simulink model "msgOutPack"  (R2023b)
settings: Solver=FixedStepDiscrete  StartTime=0.0  StopTime=10.0  FixedStep=Ts_10ms  RelTol=1e-3  EnableMultiTasking=on
values from neighbouring files (symbols this model uses):
  Ts_10ms = 0.01    [msgOutPack.sldd]
libraries: canmsglib x1
settings Model: DataDictionary=msgOutPack.sldd  Creator=62555  LastModifiedBy=62555
settings DataIOCC: SaveOutput=off  SignalLogging=off  ReturnWorkspaceOutputs=off
settings OptimizationCC: DefaultParameterBehavior=Inlined  DefaultUnderspecifiedDataType=single  EnhancedBackFolding=on  PassReuseOutputArgsAs=Individual arguments  ZeroExternalMemoryAtStartup=off  ZeroInternalMemoryAtStartup=off  OptimizeBlockOrder=speed  DifferentSizesBufferReuse=on  OptimizationCustomize=off  EfficientTunableParamExpr=on
settings DebuggingCC: ParameterTunabilityLossMsg=error
settings HardwareCC: ProdBitPerPointer=32  ProdBitPerSizeT=32  ProdBitPerPtrDiffT=32  ProdLargestAtomicInteger=Long  ProdLargestAtomicFloat=Double  ProdWordSize=32  ProdHWDeviceType=ARM Compatible->ARM Cortex-M
settings SFSimCC: MATLABDynamicMemAlloc=off
settings RTWCC: Description=Embedded Coder  SystemTargetFile=ert.tlc  GenCodeOnly=on  TemplateMakefile=ert_default_tmf  GenerateReport=on  Toolchain=MinGW64 | gmake (64-bit Windows)
settings CodeAppCC: ForceParamTrailComments=on  IgnoreCustomStorageClasses=off  OperatorAnnotations=on  SimulinkDataObjDesc=on  SFDataObjDesc=on  InsertBlockDesc=on
settings ERTTargetCC: TargetLangStandard=C99 (ISO)  SupportNonFinite=off  SupportComplex=off  ParenthesesLevel=Standards  CastingMode=Standards  InlinedParameterPlacement=NonHierarchical  ERTCustomFileTemplate=example_file_process.tlc

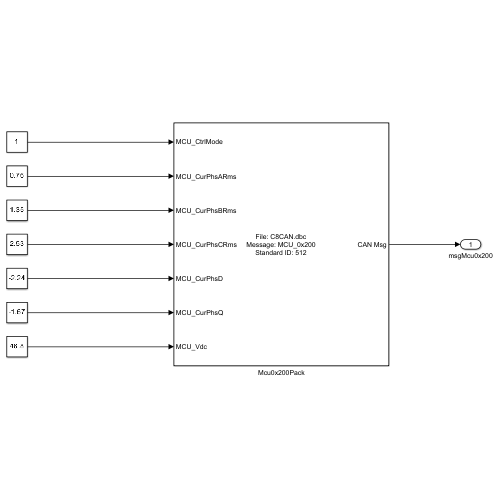
[thumbnail: Simulink's stored preview of the top-level diagram]
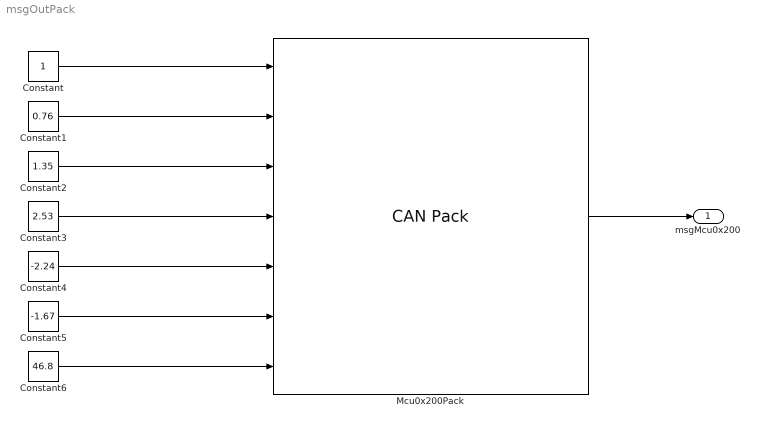
== system msgOutPack ==
  Constant : Constant  OutDataTypeStr=uint8  SampleTime=Ts_10ms
  Constant1 : Constant  Value=0.76  OutDataTypeStr=single  SampleTime=Ts_10ms
  Constant2 : Constant  Value=1.35  OutDataTypeStr=single  SampleTime=Ts_10ms
  Constant3 : Constant  Value=2.53  OutDataTypeStr=single  SampleTime=Ts_10ms
  Constant4 : Constant  Value=-2.24  OutDataTypeStr=single  SampleTime=Ts_10ms
  Constant5 : Constant  Value=-1.67  OutDataTypeStr=single  SampleTime=Ts_10ms
  Constant6 : Constant  Value=46.8  OutDataTypeStr=single  SampleTime=Ts_10ms
  Mcu0x200Pack : canmsglib/CAN Pack  CANdbFile=D:\Work\01_STM32C8CAN\03_DBC\C8CAN.dbc  MsgList=MCU_0x200  MsgName=MCU_0x200  MsgIDType=Standard (11-bit identifier)  MsgIdentifier=512  MsgLength=8  Remote=off  ApplyMinMax=off  BusOutput=off  SignalInfo={'MCU_CtrlMode','56','4','BE','unsigned','Standard','0','1','0','0','15';'MCU_CurPhsARms','14','10','BE','signed','Standard','0','0.01','0','-5.12','5.11';'MCU_CurPhsBRms','20','10','BE','signed','Standard','0','0.01','0','-5.12','5.11';'MCU_CurPhsCRms','26','10','BE','signed','Standard','0','0.01','0','-5.12','5.11';'MCU_CurPhsD','32','10','BE','signed','Standard','0','0.01','0','-5.12','5.11';'MCU_CurPhsQ','54','10','BE','signed','Standard','0','0.01','0','-5.12','5.11';'MCU_Vdc','60','10','BE','unsigned','Standard','0','0.1','0','0','102.3'}
      settings: LibrarySourceBlock=embeddedtargetslib/Host Communication/CAN Pack  DataFormat=CANdb specified signals
  msgMcu0x200 : Outport
  wires:
  Mcu0x200Pack/1 -> msgMcu0x200/1
  Constant/1 -> Mcu0x200Pack/1
  Constant1/1 -> Mcu0x200Pack/2
  Constant2/1 -> Mcu0x200Pack/3
  Constant3/1 -> Mcu0x200Pack/4
  Constant4/1 -> Mcu0x200Pack/5
  Constant5/1 -> Mcu0x200Pack/6
  Constant6/1 -> Mcu0x200Pack/7
